simulink model "ex3_sim"  (R2014b)
settings: Solver=ode45  StartTime=0.0  StopTime=5  RelTol=1e-3
values from neighbouring files (symbols this model uses):
  d = 0.5    [ex3.m]
  m = 0.1    [ex3.m]
undefined symbols (not defined in the file or in its folder): freq, G
settings Model: Creator=gabras  LastModifiedBy=gabras

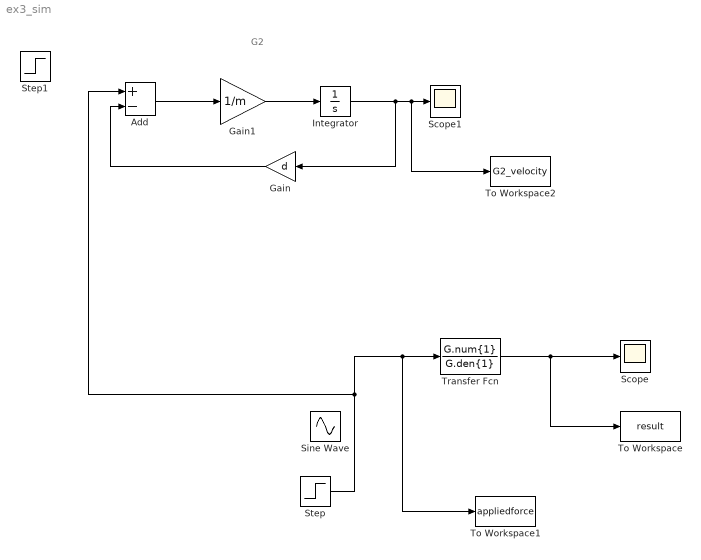
== system ex3_sim ==
  note: G2
  Add : Sum  Inputs=+-
  Gain : Gain  Gain=d
  Gain1 : Gain  Gain=1/m
  Integrator : Integrator
  Scope : Scope
      settings: YMin=-1  YMax=1
  Scope1 : Scope
  Sine Wave : Sin  Frequency=freq(1)  SampleTime=0
  Step : Step  SampleTime=0
  Step1 : Step  SampleTime=0
  To Workspace : ToWorkspace  VariableName=result  SaveFormat=Timeseries  SampleTime=-1
  To Workspace1 : ToWorkspace  VariableName=appliedforce  SaveFormat=Timeseries  SampleTime=-1
  To Workspace2 : ToWorkspace  VariableName=G2_velocity  SaveFormat=Timeseries  SampleTime=-1
  Transfer Fcn : TransferFcn  Numerator=G.num{1}  Denominator=G.den{1}
  wires:
  Transfer Fcn/1 -> To Workspace/1, Scope/1
  Step/1 -> Add/1, To Workspace1/1, Transfer Fcn/1
  Add/1 -> Gain1/1
  Gain1/1 -> Integrator/1
  Gain/1 -> Add/2
  Integrator/1 -> To Workspace2/1, Scope1/1, Gain/1
